simulink model "FanDesign"  (R2019b)
settings: Solver=VariableStepAuto  StartTime=0.0  StopTime=inf  RelTol=1e-3
settings Model: EnablePacing=on  Creator=Omer Eltayeb  LastModifiedBy=Omer Eltayeb

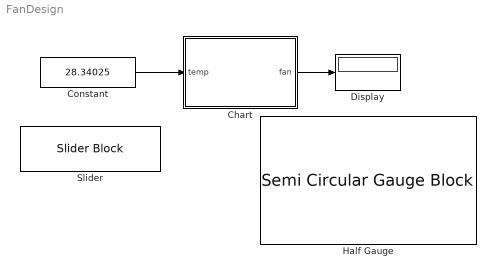
== system FanDesign ==
  Chart : Stateflow chart  BlockKeywords=__PRM__SERIALIZED__DATA__:Stateflow Chart,Stateflow Diagram  TreatAsAtomicUnit=on
  Constant : Constant  Value=28.34025
  Display : Display
  Half Gauge : SemiCircularGaugeBlock  ScaleMax=2.0
  Slider : SliderBlock  ScaleMin=1  ScaleMax=35
  wires:
  Constant/1 -> Chart/1(temp)
  Chart/1(fan) -> Display/1

== stateflow chart FanDesign/Chart ==
  state LOW
    en:
    fan=0;
  state MID
    en:
    fan=1;
  state HIGH
    en:
    fan=2;
  (default) -> LOW
  HIGH -> LOW [order 2] : [temp<18]
  LOW -> HIGH [order 2] : [temp > 25]
  LOW -> MID [order 1] : [temp>=18 && temp<=25]
  MID -> LOW [order 1] : [temp<18]
  MID -> HIGH [order 2] : [temp>25]
  HIGH -> MID [order 1] : [temp>=18 && temp <=25]
  data: temp input; fan output
